simulink model "control_mrac (2) (1) (1)"  (R2025b)
settings: Solver=VariableStepAuto  StartTime=0.0  StopTime=100  RelTol=1e-3

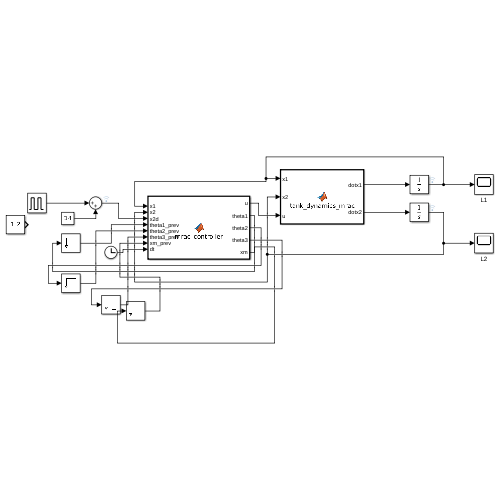
[thumbnail: Simulink's stored preview of the top-level diagram]
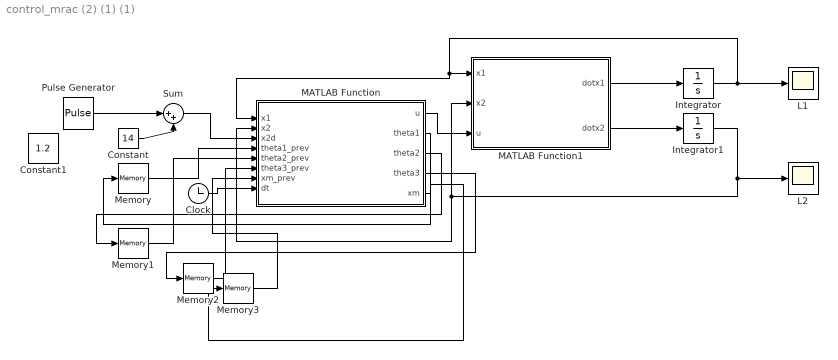
== system control_mrac (2) (1) (1) ==
  Clock : Clock
  Constant : Constant  Value=14
  Constant1 : Constant  Value=1.2
  Integrator : Integrator
  Integrator1 : Integrator
  L1 : Scope
      settings: ActiveDisplayYMinimum=-8.1372648827145362  ActiveDisplayYMaximum=8.6893327676980583
  L2 : Scope
      settings: ActiveDisplayYMinimum=-4.3997183929436492  ActiveDisplayYMaximum=20.189488092755962
  MATLAB Function : MATLAB Function  TreatAsAtomicUnit=on
  MATLAB Function1 : MATLAB Function  TreatAsAtomicUnit=on
  Memory{,1..3} (4 alike) : Memory  InitialCondition=0.5
  Pulse Generator : DiscretePulseGenerator  PulseType=Time based  Amplitude=2  Period=20  PulseWidth=50
  Sum : Sum  Inputs=|++
  wires:
  Integrator1/1 -> L2/1, MATLAB Function1/2(x2), MATLAB Function/2(x2)
  Pulse Generator/1 -> Sum/1
  Constant/1 -> Sum/2
  Integrator/1 -> L1/1, MATLAB Function1/1(x1), MATLAB Function/1(x1)
  MATLAB Function1/1(dotx1) -> Integrator/1
  MATLAB Function1/2(dotx2) -> Integrator1/1
  Sum/1 -> MATLAB Function/3(x2d)
  MATLAB Function/1(u) -> MATLAB Function1/3(u)
  MATLAB Function/2(theta1) -> Memory/1
  Memory/1 -> MATLAB Function/4(theta1_prev)
  MATLAB Function/3(theta2) -> Memory1/1
  Memory1/1 -> MATLAB Function/5(theta2_prev)
  MATLAB Function/4(theta3) -> Memory2/1
  Memory2/1 -> MATLAB Function/6(theta3_prev)
  MATLAB Function/5(xm) -> Memory3/1
  Memory3/1 -> MATLAB Function/7(xm_prev)
  Clock/1 -> MATLAB Function/8(dt)

== matlab function control_mrac (2) (1) (1)/MATLAB Function1 ==
  data: x1 input; x2 input; u input; dotx1 output; dotx2 output
function [dotx1, dotx2] = tank_dynamics_mrac(x1, x2, u)
% TANK_DYNAMICS_MRAC - Dinámica de tanques para control MRAC

% PARÁMETROS DEL SISTEMA (consistentes con el controlador)
a1 = 1.1513;    % cm^{1/2}/s
a2 = 0.6467;    % cm^{1/2}/s
b1 = 0.2126;    % cm/s/V

% Asegurar que los niveles sean no negativos
x1_safe = max(x1, 0.001);
x2_safe = max(x2, 0.001);

% Ecuaciones de estado
dotx1 = -a1 * sqrt(x1_safe) + b1 * u;
dotx2 = a1 * sqrt(x1_safe) - a2 * sqrt(x2_safe);
end

== matlab function control_mrac (2) (1) (1)/MATLAB Function ==
  data: x1 input; u output; x2 input; x2d input; theta1_prev input; theta2_prev input; theta3_prev input; xm_prev input; dt input; theta1 output; theta2 output; theta3 output; xm output
function [u, theta1, theta2, theta3, xm] = mrac_controller(...
    x1, x2, x2d, theta1_prev, theta2_prev, theta3_prev, xm_prev, dt)
%#codegen

% Especificar dimensiones de salida
u = zeros(1, 1);           % Salida escalar [1x1]
theta1 = zeros(1, 1);      % Parámetro escalar [1x1]
theta2 = zeros(1, 1);      % Parámetro escalar [1x1]  
theta3 = zeros(1, 1);      % Parámetro escalar [1x1]
xm = zeros(2, 1);          % Vector de estado [2x1]

% PARÁMETROS DEL SISTEMA
a1 = 1.1513;    % cm^{1/2}/s
a2 = 0.6467;    % cm^{1/2}/s  
b1 = 0.2126;    % cm/s/V

% PARÁMETROS MRAC
omega_n = 1.5;  zeta = 0.8;  gamma = 0.5;

% Asegurar valores positivos
x1_safe = max(x1, 0.001);
x2_safe = max(x2, 0.001);

% Modelo de referencia (segundo orden)
Am = [0, 1; -omega_n^2, -2*zeta*omega_n];
Bm = [0; omega_n^2];

% Integrar modelo de referencia
xm_dot = Am * xm_prev + Bm * x2d;
xm = xm_prev + xm_dot * dt;

% Error de seguimiento
e = x2_safe - xm(1);

% Vector de regresión
phi = [x2_safe; x1_safe; x2d];

% Ley de control MRAC
u = theta1_prev * x2_safe + theta2_prev * x1_safe + theta3_prev * x2d;

% Ley de adaptación
theta_dot = -gamma * e * phi;
theta1 = theta1_prev + theta_dot(1) * dt;
theta2 = theta2_prev + theta_dot(2) * dt;
theta3 = theta3_prev + theta_dot(3) * dt;

% Saturación
u = max(0, min(u, 12));
end
